simulink model "V3_sim"  (R2017a)
settings: Solver=ode45  StartTime=0.0  StopTime=Te  RelTol=1e-10  EnableMultiTasking=on
InitFcn:
  | initScript;
values from neighbouring files (symbols this model uses):
  M_AP = []    [V3_initSim.m]    (also in initScript.m = 0)
  stPendel = ladePendel()    [V3_initSim.m]    (also in initScript.m; simGUI.m; test_bvp4c.m)
  x0 = [-pi/3 0 pi 0]    [V3_initSim.m]    (also in initScript.m = [0 0 0 0])
settings Model: Creator=bened  LastModifiedBy=bened
settings OptimizationCC: LifeSpan=inf
settings DebuggingCC: SFUnexpectedBacktrackingDiag=warning  SFNoUnconditionalDefaultTransitionDiag=warning  SFExecutionAtInitializationDiag=none
settings GRTTargetCC: TargetLangStandard=C89/C90 (ANSI)
settings ConfigComp: CovMetricSettings=dw  CovHtmlReporting=on  CovSaveCumulativeToWorkspaceVar=on  CovSaveSingleToWorkspaceVar=on  CovExternalEMLEnable=off

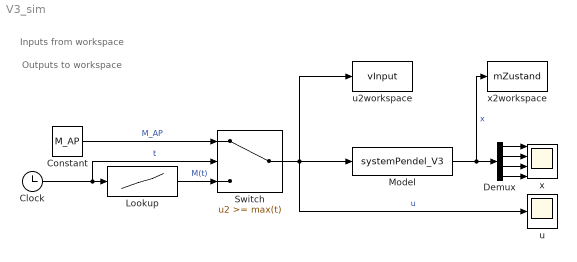
== system V3_sim ==
  note: Inputs from workspace
  note: Outputs to workspace
  Clock : Clock
  Constant : Constant  Value=M_AP
  Demux : Demux
  "Lookup " : Lookup_n-D  NumberOfTableDimensions=1  LookupTableObject=lut  BreakpointsForDimension1=t  BreakpointsForDimension2=[1:3]  Table=u  InterpMethod=Cubic spline  ExtrapMethod=Clip  InternalRulePriority=Speed  RndMeth=Simplest  InputSameDT=on
  Model : M-S-Function  FunctionName=systemPendel_V3  Parameters=stPendel,x0
  Switch : Switch  Threshold=max(t)
  "u " : Scope
  u2workspace : ToWorkspace  VariableName=vInput  SaveFormat=Structure With Time  SampleTime=-1
  x : Scope  NumInputPorts=4
  x2workspace : ToWorkspace  VariableName=mZustand  SaveFormat=Structure With Time  SampleTime=-1
  wires:
  Model/1 -> x2workspace/1, Demux/1  "x"
  Switch/1 -> "u "/1, Model/1, u2workspace/1  "u"
  Demux/1 -> x/1
  Demux/2 -> x/2
  Demux/3 -> x/3
  Demux/4 -> x/4
  Clock/1 -> Switch/2, "Lookup "/1  "t"
  "Lookup "/1 -> Switch/3  "M(t)"
  Constant/1 -> Switch/1  "M_AP"
